simulink model "sm_boom_lift_crawler_abstract_flex_boom"  (R2026a)
settings: Solver=ode23t  StopTime=operator_seq.StopTime  FixedStep=2e-2  MaxStep=2  AbsTol=1e-3
PreLoadFcn:
  | sm_boom_lift_crawler_settest('full test')
StartFcn:
  | tic;
StopFcn:
  | Elapsed_Sim_Time = toc;
  | %disp(['Elapsed Sim Time = ' num2str(Elapsed_Sim_Time)]);
undefined symbols (not defined in the file or in its folder): b, BasketR, Boom, Chassis, Extend, FL, FR, Jib, LevelM, LevelS, Lift, operator_seq, OutFL, OutFR, OutRL, OutRR, RL, RR, Tilt, TrackL, TrackR, Turret, X, Y, Z
libraries: sm_lib x67, sm_boom_lift_crawler_lib x22, nesl_utility x15, sm_boom_lift_crawler_lib_boom x5, sm_boom_lift_crawler_lib_control x1, sm_boom_lift_crawler_lib_chassis x1
(part 1 of 5)
Description:
  | Boom Lift Crawler with Flexible Boom
  | 
  | Copyright 2020-2026 The MathWorks, Inc.
settings Model: PacingRate=0.100000  Creator=smiller  LastModifiedBy=smiller
settings DataIOCC: SignalLoggingName=logsout_sm_boom_lift_crawler
settings SimscapeCC: SimscapeNominalValues="[{\"value\":\"1\",\"unit\":\"A\"},{\"value\":\"nomval_psi\",\"unit\":\"psi\"},{\"value\":\"1\",\"unit\":\"cm^2\"},{\"value\":\"nomval_cmv3_s\",\"unit\":\"cm^3/s\"},{\"value\":\"1\",\"unit\":\"kJ/kg\"},{\"value\":\"1\",\"unit\":\"kW\"},{\"value\":\"1\",\"unit\":\"l\"},{\"value\":\"nomval_N\",\"unit\":\"N\"},{\"value\":\"nomval_Nm\",\"unit\":\"N*m\"},{\"value\":\"1\",\"unit\":\"V\"}]"  SimscapeLogName=simlog_sm_boom_lift_crawler  SimscapeLogLimitData=off  SimscapeLogDataHistory=5000.0  SimscapeOperatingPoint=op_hold15Sec_FULL
settings DiagnosticsConfigSet: SimMechanicsConflictingReferenceFrames=none  SimMechanicsRigidlyBoundBlock=none
settings ExplorerConfigSet: InternalSimMechanicsExplorerSettings="<ExplorerConfiguration><canonicalview>default</canonicalview><AnimationSetting><BasePlaybackSpeed>1.0</BasePlaybackSpeed><PlaybackSpeedFactor>1.0</PlaybackSpeedFactor></AnimationSetting><TilePanel><TileInfo><Tiles Columns=\"2\" Count=\"2\" Rows=\"1\"><Column Weight=\"0.4\"/><Column Weight=\"0.6\"/><Row Weight=\"1\"/><Tile Height=\"1\" Width=\"1\" X=\"0\" Y=\"0\"/><Tile Height=\"1\" Width=\"1\" X=\"1\" Y=\"0\"/></Tiles></TileInfo><SceneInfo><SceneViewer><BGColor><R>1</R><G>1</G><B>1</B></BGColor><Camera><DoPerspective>on</DoPerspective><Position><X>0.861797228389737158</X><Y>15.4087919652116785</Y><Z>1.5985929178525955</Z></Position><Center><X>0.688433827393987063</X><Y>14.4239340408412708</Y><Z>1.59859291785259594</Z></Center><Up><X>0</X><Y>0</Y><Z>1</Z></Up><ViewLimDist>1</ViewLimDist><YLim>0.466307658154998583</YLim><XLim>0.206102832333701025</XLim></Camera></SceneViewer><SceneViewer><BGColor><R>1</R><G>1</G><B>1</B></BGColor><Camera><DoPerspective>off</DoPerspective><Position><X>-13.0744225167074219</X><Y>9.83182144578760031</Y><Z>7.16198046954759793</Z></Position><Center><X>1.63071735726949996</X><Y>4.41437199856754514</Y><Z>7.1529177327451432</Z></Center><Up><X>0</X><Y>0</Y><Z>1</Z></Up><ViewLimDist>1</ViewLimDist><YLim>15.4925512172975477</YLim><XLim>10.3283674781983645</XLim></Camera></SceneViewer></SceneInfo></TilePanel><MechEditorPanel><Cameras><Camera><Id>Camera8</Id><Value><Name>Extend_Knuckle</Name><NativeCamera><PositionTrackingFeature>Lift.Boom.Arms.Telescope.Extend_Cylinder.Transform_Camera_Extend_Knuckle.F</PositionTrackingFeature><CenterTrackingFeature>Lift.Boom.Arms.Telescope.Extend_Cylinder.Transform_Camera_Extend_Knuckle.F</CenterTrackingFeature><UpVectorTrackingFeature>Lift.Boom.Arms.Telescope.Extend_Cylinder.Transform_Camera_Extend_Knuckle.F</UpVectorTrackingFeature><CenterTrackingOrigin>off</CenterTrackingOrigin><CenterTrackingDirection>-X</CenterTrackingDirection><UpVectorTrackingDirection>-Y</UpVectorTrackingDirection></NativeCamera></Value></Camera><Camera><Id>Camera9</Id><Value><Name>Extend_Basket</Name><NativeCamera><PositionTrackingFeature>Lift.Boom.Arms.Telescope.Extend_Cylinder.Transform_Camera_Extend_Basket.F</PositionTrackingFeature><CenterTrackingFeature>Lift.Boom.Arms.Telescope.Extend_Cylinder.Transform_Camera_Extend_Basket.F</CenterTrackingFeature><UpVectorTrackingFeature>Lift.Boom.Arms.Telescope.Extend_Cylinder.Transform_Camera_Extend_Basket.F</UpVectorTrackingFeature><CenterTrackingOrigin>off</CenterTrackingOrigin><CenterTrackingDirection>+X</CenterTrackingDirection><UpVectorTrackingDirection>+Y</UpVectorTrackingDirection></NativeCamera></Value></Camera><Camera><Id>Camera10</Id><Value><Name>Basket_Rotate</Name><NativeCamera><PositionTrackingFeature>Lift.Boom.Basket.Basket_Rotate.Bracket.Reference_Camera_Basket_Rotate_L.R</PositionTrackingFeature><CenterTrackingFeature>Lift.Boom.Basket.Basket_Rotate.Bracket.Reference_Camera_Basket_Rotate_L.R</CenterTrackingFeature><UpVectorTrackingFeature>Mech_Config.World.W</UpVectorTrackingFeature><CenterTrackingOrigin>off</CenterTrackingOrigin><CenterTrackingDirection>-X</CenterTrackingDirection><UpVectorTrackingDirection>+Z</UpVectorTrackingDirection></NativeCamera></Value></Camera><Camera><Id>Camera11</Id><Value><Name>Tilt_Knuckle</Name><NativeCamera><PositionTrackingFeature>Lift.Boom.Arms.Tower.Upper_Knuckle.Reference_Knuckle_Cam.R</PositionTrackingFeature><CenterTrackingFeature>Lift.Boom.Arms.Tower.Upper_Knuckle.Reference_Knuckle_Cam.R</CenterTrackingFeature><UpVectorTrackingFeature>Mech_Config.World.W</UpVectorTrackingFeature><CenterTrackingOrigin>off</CenterTrackingOrigin><CenterTrackingDirection>+Z</CenterTrackingDirection><UpVectorTrackingDirection>+Z</UpVectorTrackingDirection></NativeCamera></Value></Camera><Camera><Id>Camera12</Id><Value><Name>Full Test</Name><NativeCamera><PositionKeyframeSet><Keyframe><Time>0</Time><Value><X>-12.242458171438994</X><Y>-0.1433452642095574</Y><Z>4.1505972342390427</Z></Value></Keyframe><Keyframe><Time>69.026826430124729</Time><Value><X>-14.974593328379619</X><Y>0.0056652615564253064</Y><Z>5.3389029552684786</Z></Value></Keyframe><Keyframe><Time>110.29539843687829</Time><Value><X>-21.00761369699504</X><Y>-0.0057417156870510078</Y><Z>8.0689402037867488</Z></Value></Keyframe><Keyframe><Time>140.70430157635164</Time><Value><X>-31.272784439198116</X><Y>-2.5583130214499052e-10</Y><Z>12.723321478963756</Z></Value></Keyframe><Keyframe><Time>181.77628976806102</Time><Value><X>-31.272784439198116</X><Y>-2.5583130214499052e-10</Y><Z>12.723321478963756</Z></Value></Keyframe><Keyframe><Time>208.0087867386398</Time><Value><X>-23.351505250921551</X><Y>-2.5583182919801497e-10</Y><Z>9.1371534281977738</Z></Value></Keyframe><Keyframe><Time>243.06358572448306</Time><Value><X>-16.577121762622586</X><Y>-2.5583144573665537e-10</Y><Z>6.0702143126734844</Z></Value></Keyframe><Keyframe><Time>273.3415757110605</Time><Value><X>-16.577121762622586</X><Y>-2.5583144573665537e-10</Y><Z>6.0702143126734844</Z></Value></Keyframe><Keyframe><Time>321.2447002217541</Time><Value><X>-13.690590902490033</X><Y>0.01787769923724114</Y><Z>4.7891626503614262</Z></Value></Keyframe><Keyframe><Time>350</Time><Value><X>-13.690590902490033</X><Y>0.01787769923724114</Y><Z>4.7891626503614262</Z></Value></Keyframe></PositionKeyframeSet><CenterKeyframeSet><Keyframe><Time>0</Time><Value><X>-4.621228999686064</X><Y>-0.1433452642095574</Y><Z>4.1505972342390436</Z></Value></Keyframe><Keyframe><Time>69.026826430124729</Time><Value><X>-0.17395018713353672</X><Y>0.0056652615564253064</Y><Z>5.3389029552684786</Z></Value></Keyframe><Keyframe><Time>110.29539843687829</Time><Value><X>-9.0038066291239502</X><Y>-0.0057417156870549491</Y><Z>8.0689402037867524</Z></Value></Keyframe><Keyframe><Time>140.70430157635164</Time><Value><X>-14.136391845814327</X><Y>-2.5583979379462107e-10</Y><Z>12.72332147896376</Z></Value></Keyframe><Keyframe><Time>181.77628976806102</Time><Value><X>-2.3429975002054775</X><Y>-2.5584563781180217e-10</Y><Z>12.723321478963761</Z></Value></Keyframe><Keyframe><Time>208.0087867386398</Time><Value><X>-10.17575261115104</X><Y>-2.5583801743778167e-10</Y><Z>9.1371534281977755</Z></Value></Keyframe><Keyframe><Time>243.06358572448306</Time><Value><X>-0.54476849060194255</X><Y>-2.5583897563257738e-10</Y><Z>6.0702143126734844</Z></Value></Keyframe><Keyframe><Time>273.3415757110605</Time><Value><X>-0.11057247639663359</X><Y>-2.5583917956089291e-10</Y><Z>6.0702143126734844</Z></Value></Keyframe><Keyframe><Time>321.2447002217541</Time><Value><X>-5.3452949964231387</X><Y>0.017877699237237366</Y><Z>4.7891626503614253</Z></Value></Keyframe><Keyframe><Time>350</Time><Value><X>-5.3452949964231387</X><Y>0.017877699237237366</Y><Z>4.7891626503614253</Z></Value></Keyframe></CenterKeyframeSet><UpVectorKeyframeSet><Keyframe><Time>0</Time><Value><X>0</X><Y>0</Y><Z>1</Z></Value></Keyframe><Keyframe><Time>69.026826430124729</Time><Value><X>0</X><Y>0</Y><Z>1</Z></Value></Keyframe><Keyframe><Time>110.29539843687829</Time><Value><X>0</X><Y>0</Y><Z>1</Z></Value></Keyframe><Keyframe><Time>140.70430157635164</Time><Value><X>0</X><Y>0</Y><Z>1</Z></Value></Keyframe><Keyframe><Time>181.77628976806102</Time><Value><X>-2.0731981129868445e-16</X><Y>1.0273382740432149e-31</Y><Z>1</Z></Value></Keyframe><Keyframe><Time>208.0087867386398</Time><Value><X>1.4663775813922931e-57</X><Y>2.9591920320379324e-42</Y><Z>1</Z></Value></Keyframe><Keyframe><Time>243.06358572448306</Time><Value><X>1.3898401336634517e-57</X><Y>2.9591920320379324e-42</Y><Z>1</Z></Value></Keyframe><Keyframe><Time>273.3415757110605</Time><Value><X>1.3898401336605064e-57</X><Y>2.9591920320379324e-42</Y><Z>1</Z></Value></Keyframe><Keyframe><Time>321.2447002217541</Time><Value><X>1.3198478700492623e-57</X><Y>2.9591920320379324e-42</Y><Z>1</Z></Value></Keyframe><Keyframe><Time>350</Time><Value><X>1.0642863113510858e-16</X><Y>-4.813997747953607e-32</Y><Z>1</Z></Value></Keyframe></UpVectorKeyframeSet></NativeCamera></Value></Camera><Camera><Id>Camera13</Id><Value><Name>View_Basket_World</Name><NativeCamera><PositionTrackingFeature>Lift.Boom.Basket.Basket.Reference_Basket_Cam.R</PositionTrackingFeature><CenterTrackingFeature>Mech_Config.World.W</CenterTrackingFeature><UpVectorTrackingFeature>Lift.Boom.Basket.Basket.Reference_Basket_Cam.R</UpVectorTrackingFeature><CenterTrackingOrigin>on</CenterTrackingOrigin><UpVectorTrackingDirection>+Y</UpVectorTrackingDirection></NativeCamera></Value></Camera><Camera><Id>Camera14</Id><Value><Name>View_Worm_Drive</Name><NativeCamera><PositionTrackingFeature>Lift.Boom.Turret.Case.Reference_Worm_Cam.R</PositionTrackingFeature><CenterTrackingFeature>Lift.Boom.Turret.Case.Transform_Worm_Cam.B</CenterTrackingFeature><UpVectorTrackingFeature>Mech_Config.World.W</UpVectorTrackingFeature><CenterTrackingOrigin>on</CenterTrackingOrigin><UpVectorTrackingDirection>+Z</UpVectorTrackingDirection></NativeCamera></Value></Camera><Camera><Id>Camera15</Id><Value><Name>Extend_Retract_Pulley</Name><NativeCamera><PositionTrackingFeature>Lift.Boom.Arms.Telescope.Extend_Cylinder.Reference_Camera_Retract_Pulley.R</PositionTrackingFeature><CenterTrackingFeature>Lift.Boom.Arms.Telescope.Extend_Cylinder.Reference_Camera_Retract_Pulley.R</CenterTrackingFeature><UpVectorTrackingFeature>Lift.Boom.Arms.Telescope.Extend_Cylinder.Reference_Camera_Retract_Pulley.R</UpVectorTrackingFeature><CenterTrackingOrigin>off</CenterTrackingOrigin><CenterTrackingDirection>+Y</CenterTrackingDirection><UpVectorTrackingDirection>+Z</UpVectorTrackingDirection></NativeCamera></Value></Camera><Camera><Id>Camera16</Id><Value><Name>Extend_Extend_Pulley</Name><NativeCamera><PositionTrackingFeature>Lift.Boom.Arms.Telescope.Extend_Cylinder.Reference_Camera_Extend_Pulley.R</PositionTrackingFeature><CenterTrackingFeature>Lift.Boom.Arms.Telescope.Extend_Cylinder.Reference_Camera_Extend_Pulley.R</CenterTrackingFeature><UpVectorTrackingFeature>Lift.Boom.Arms.Telescope.Extend_Cylinder.Reference_Camera_Extend_Pulley.R</UpVectorTrackingFeature><CenterTrackingOrigin>off</CenterTrackingOrigin><CenterTrackingDirection>+Z</CenterTrackingDirection><UpVectorTrackingDirection>-Y</UpVectorTrackingDirection></NativeCamera></Value></Camera><Camera><Id>Camera17</Id><Value><Name>Jib</Name><NativeCamera><PositionTrackingFeature>Lift.Boom.Basket.Jib.Jib_Mount.Reference_Camera_Basket_Jib.R</PositionTrackingFeature><CenterTrackingFeature>Lift.Boom.Basket.Jib.Jib_Mount.Reference_Camera_Basket_Jib.R</CenterTrackingFeature><UpVectorTrackingFeature>Mech_Config.World.W</UpVectorTrackingFeature><CenterTrackingOrigin>off</CenterTrackingOrigin><CenterTrackingDirection>-X</CenterTrackingDirection><UpVectorTrackingDirection>+Z</UpVectorTrackingDirection></NativeCamera></Value></Camera><Camera><Id>Camera18</Id><Value><Name>Boom Align</Name><NativeCamera><PositionTrackingFeature>Lift.Chassis.Frame.Reference_Camera_Boom_Align_R</PositionTrackingFeature><CenterTrackingFeature>Lift.Chassis.Frame.Reference_Camera_Boom_Align_R</CenterTrackingFeature><UpVectorTrackingFeature>Lift.Chassis.Frame.Reference_Camera_Boom_Align_R</UpVectorTrackingFeature><CenterTrackingOrigin>off</CenterTrackingOrigin><CenterTrackingDirection>+Y</CenterTrackingDirection><UpVectorTrackingDirection>+Z</UpVectorTrackingDirection></NativeCamera></Value></Camera><Camera><Id>Camera19</Id><Value><Name>Basket_Boom</Name><NativeCamera><PositionTrackingFeature>Lift.Boom.Arms.Camera_Boom_Basket.Reference_Basket_Boom_Cam.R</PositionTrackingFeature><CenterTrackingFeature>Lift.Boom.Arms.Camera_Boom_Basket.Reference_Basket_Boom_Cam.R</CenterTrackingFeature><UpVectorTrackingFeature>Mech_Config.World.W</UpVectorTrackingFeature><CenterTrackingOrigin>off</CenterTrackingOrigin><CenterTrackingDirection>+X</CenterTrackingDirection><UpVectorTrackingDirection>+Z</UpVectorTrackingDirection></NativeCamera></Value></Camera></Cameras><GfxPanelCameraMap><MapElement CameraMLId=\"Camera19\" GfxPanelIndex=\"0\"/></GfxPanelCameraMap><VideoCreator><PlaybackSpeedRatio>1.0</PlaybackSpeedRatio><FrameRate>30</FrameRate><VideoFormat>MPEG-4</VideoFormat><FrameSize>auto</FrameSize></VideoCreator></MechEditorPanel></ExplorerConfiguration>"

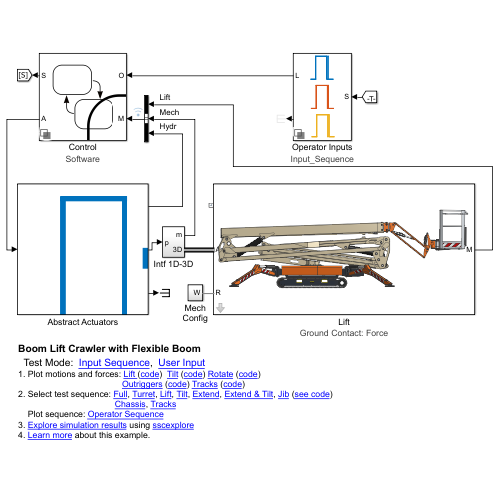
[thumbnail: Simulink's stored preview of the top-level diagram]
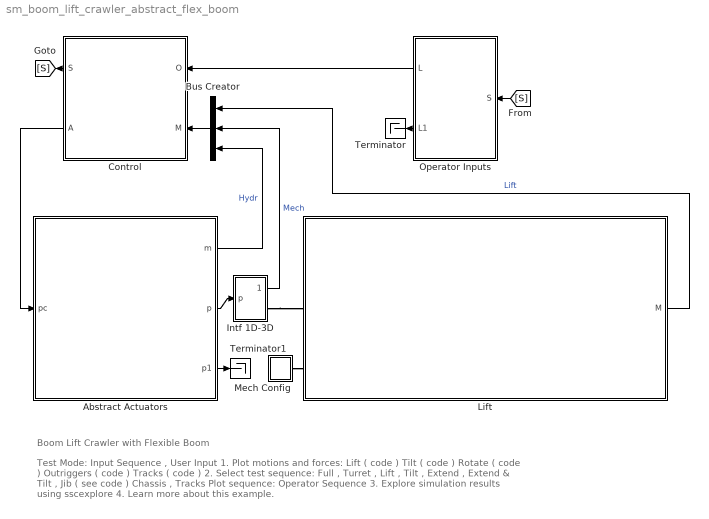
== system sm_boom_lift_crawler_abstract_flex_boom ==
  note: Test Mode: Input Sequence , User Input
      | 1. Plot motions and forces: Lift ( code ) Tilt ( code ) Rotate ( code )
      | Outriggers ( code ) Tracks ( code )
      | 2. Select test sequence: Full , Turret , Lift , Tilt , Extend , Extend & Tilt , Jib ( see code )
      | Chassis , Tracks
      | Plot sequence: Operator Sequence
      | 3. Explore simulation results using sscexplore
      | 4. Learn more about this example.
  note: Boom Lift Crawler with Flexible Boom
  Abstract Actuators : Subsystem  VariantControl=Controller_Inputs
      mask Display: image('sm_boom_lift_crawler_logic_to_motion_seq.svg');
  Bus Creator : BusCreator  Inputs=3
  Control : Subsystem  Variant=on  VariantControlMode=label  VariantControl=Variant1  LabelModeActiveChoice=Software
      settings: AttributesFormatString=%<LabelModeActiveChoice>
      mask Display:
      | blk = sm_boom_lift_activeVariantBlock(gcb);
      | eval(get_param(blk, 'MaskDisplay'));
  Intf 1D-3D : Subsystem
  Lift : Subsystem  mask{popup_gnd_outr=Force}
      mask prompts: popup_gnd_outr "Ground Contact (Outrigger)"
      mask init:
      | set_param([gcb '/Ground Contact Pads'],'LabelModeActiveChoice',get_param(gcb,'popup_gnd_outr'));
      settings: AttributesFormatString=Ground Contact: %<popup_gnd_outr>
      mask TypeOptions popup_gnd_outr: Force | Constraint
      mask Display: image('sm001_2x1_v2.svg');
  Mech Config : Subsystem
  Operator Inputs : Subsystem  Variant=on  VariantControlMode=label  VariantControl=Variant1  LabelModeActiveChoice=Input_Sequence
      settings: AttributesFormatString=%<LabelModeActiveChoice>
      mask Display:
      | blk = sm_boom_lift_activeVariantBlock(gcb);
      | eval(get_param(blk, 'MaskDisplay'));
  Terminator : Terminator
  Terminator1 : Terminator
  wires:
  Intf 1D-3D/1(m) -> Bus Creator/2  "Mech"
  Bus Creator/1 -> Control/2(M)
  Lift/1(M) -> Bus Creator/1  "Lift"
  Control/2(A) -> Abstract Actuators/1(pc)
  Abstract Actuators/2(p) -> Intf 1D-3D/1(p)
  Abstract Actuators/3(p1) -> Terminator1/1
  Abstract Actuators/1(m) -> Bus Creator/3  "Hydr"
  Operator Inputs/1(L) -> Control/1(O)
  Operator Inputs/2(L1) -> Terminator/1
  Control/1(S) -> [S]
  [S] -> Operator Inputs/1(S)
  connections:
  Mech Config/LConn1 -- Lift/LConn3
  Intf 1D-3D/RConn1 -- Lift/LConn2

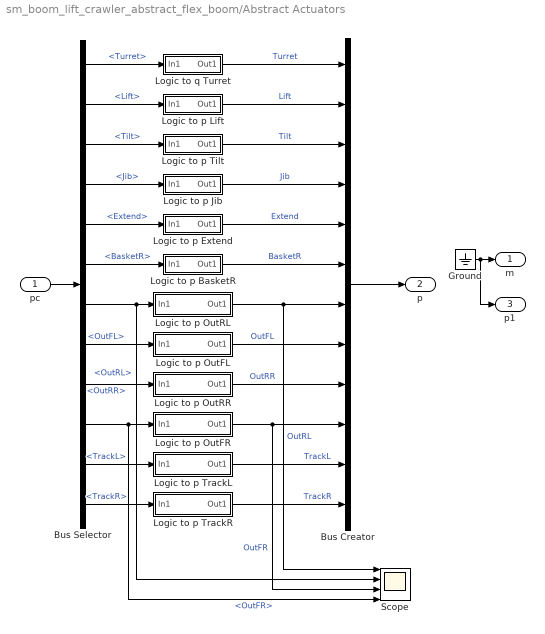
== system sm_boom_lift_crawler_abstract_flex_boom/Abstract Actuators ==
  pc : Inport
  Bus Creator : BusCreator  Inputs=12
  Bus Selector : BusSelector  OutputSignals=Turret,Lift,Tilt,Jib,Extend,BasketR,OutRL,OutFL,OutRR,OutFR,TrackL,TrackR
  Ground : Ground
  Logic to p BasketR : Subsystem
  Logic to p Extend : Subsystem
  Logic to p Jib : Subsystem
  Logic to p Lift : Subsystem
  Logic to p OutFL : Subsystem
  Logic to p OutFR : Subsystem
  Logic to p OutRL : Subsystem
  Logic to p OutRR : Subsystem
  Logic to p Tilt : Subsystem
  Logic to p TrackL : Subsystem
  Logic to p TrackR : Subsystem
  Logic to q Turret : Subsystem
  Scope : Scope  NumInputPorts=4
      settings: ActiveDisplayYMinimum=12.92005  ActiveDisplayYMaximum=13.76598
  m : Outport
  p : Outport  Port=2
  p1 : Outport  Port=3
  wires:
  Ground/1 -> m/1, p1/1
  pc/1 -> Bus Selector/1
  Bus Selector/12 -> Logic to p TrackR/1(In1)  "<TrackR>"
  Bus Selector/11 -> Logic to p TrackL/1(In1)  "<TrackL>"
  Bus Selector/2 -> Logic to p Lift/1(In1)  "<Lift>"
  Logic to p TrackL/1(Out1) -> Bus Creator/11  "TrackL"
  Bus Selector/6 -> Logic to p BasketR/1(In1)  "<BasketR>"
  Bus Selector/5 -> Logic to p Extend/1(In1)  "<Extend>"
  Bus Creator/1 -> p/1
  Bus Selector/1 -> Logic to q Turret/1(In1)  "<Turret>"
  Bus Selector/7 -> Scope/2, Logic to p OutRL/1(In1)  "<OutRL>"
  Bus Selector/3 -> Logic to p Tilt/1(In1)  "<Tilt>"
  Logic to p Lift/1(Out1) -> Bus Creator/2  "Lift"
  Bus Selector/8 -> Logic to p OutFL/1(In1)  "<OutFL>"
  Bus Selector/4 -> Logic to p Jib/1(In1)  "<Jib>"
  Logic to p TrackR/1(Out1) -> Bus Creator/12  "TrackR"
  Bus Selector/9 -> Logic to p OutRR/1(In1)  "<OutRR>"
  Bus Selector/10 -> Scope/4, Logic to p OutFR/1(In1)  "<OutFR>"
  Logic to q Turret/1(Out1) -> Bus Creator/1  "Turret"
  Logic to p OutRL/1(Out1) -> Scope/1, Bus Creator/7  "OutRL"
  Logic to p OutFL/1(Out1) -> Bus Creator/8  "OutFL"
  Logic to p OutRR/1(Out1) -> Bus Creator/9  "OutRR"
  Logic to p OutFR/1(Out1) -> Scope/3, Bus Creator/10  "OutFR"
  Logic to p Tilt/1(Out1) -> Bus Creator/3  "Tilt"
  Logic to p Jib/1(Out1) -> Bus Creator/4  "Jib"
  Logic to p Extend/1(Out1) -> Bus Creator/5  "Extend"
  Logic to p BasketR/1(Out1) -> Bus Creator/6  "BasketR"

== system sm_boom_lift_crawler_abstract_flex_boom/Control ==
  O : Inport
  M : Inport  Port=2
  Direct : Subsystem  VariantControl=Direct
      mask Display: image('sm_boom_lift_crawler_control_direct.svg');
  Software : sm_boom_lift_crawler_lib_control/Software  SystemSampleTime=-1  VariantControl=Software  VariantActivationTime=update diagram  EmptyChoice=off  PassThrough=off  PassThroughVariantControl=(default)  EmptyChoiceVariantControl=(default)  AllowFlexibleInterface=on  Latency=0  AutoFrameSizeCalculation=off
  S : Outport
  A : Outport  Port=2

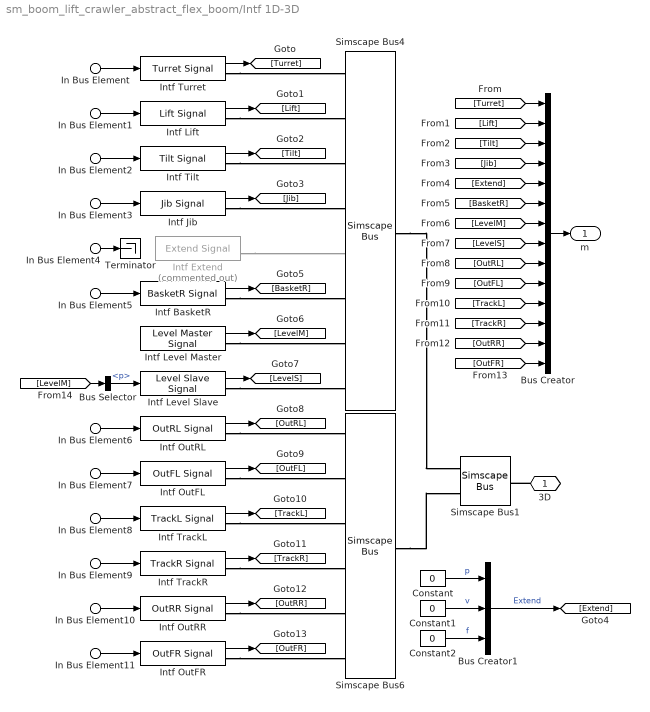
== system sm_boom_lift_crawler_abstract_flex_boom/Intf 1D-3D ==
  In Bus Element : Inport  PortName=p  Element=Turret
  In Bus Element1 : Inport  PortName=p  Element=Lift
  In Bus Element2 : Inport  PortName=p  Element=Tilt
  In Bus Element3 : Inport  PortName=p  Element=Jib
  In Bus Element4 : Inport  PortName=p  Element=Extend
  In Bus Element5 : Inport  PortName=p  Element=BasketR
  In Bus Element6 : Inport  PortName=p  Element=OutRL
  In Bus Element7 : Inport  PortName=p  Element=OutFL
  In Bus Element8 : Inport  PortName=p  Element=TrackL
  In Bus Element9 : Inport  PortName=p  Element=TrackR
  In Bus Element10 : Inport  PortName=p  Element=OutRR
  In Bus Element11 : Inport  PortName=p  Element=OutFR
  Bus Creator : BusCreator  Inputs=14
  Bus Creator1 : BusCreator  Inputs=3
  Bus Selector : BusSelector  OutputSignals=p
  Constant : Constant  Value=0
  Constant1 : Constant  Value=0
  Constant2 : Constant  Value=0
  Intf BasketR : sm_boom_lift_crawler_lib/BasketR Signal  SystemSampleTime=-1  VariantActivationTime=update diagram  EmptyChoice=off  PassThrough=off  PassThroughVariantControl=(default)  EmptyChoiceVariantControl=(default)  AllowFlexibleInterface=on  Latency=0  AutoFrameSizeCalculation=off
  Intf Extend : sm_boom_lift_crawler_lib/Extend Signal  Commented=on  SystemSampleTime=-1  VariantActivationTime=update diagram  EmptyChoice=off  PassThrough=off  PassThroughVariantControl=(default)  EmptyChoiceVariantControl=(default)  AllowFlexibleInterface=on  Latency=0  AutoFrameSizeCalculation=off
  Intf Jib : sm_boom_lift_crawler_lib/Jib Signal  SystemSampleTime=-1  VariantActivationTime=update diagram  EmptyChoice=off  PassThrough=off  PassThroughVariantControl=(default)  EmptyChoiceVariantControl=(default)  AllowFlexibleInterface=on  Latency=0  AutoFrameSizeCalculation=off
  Intf Level Master : sm_boom_lift_crawler_lib/Level Master Signal  SystemSampleTime=-1  VariantActivationTime=update diagram  EmptyChoice=off  PassThrough=off  PassThroughVariantControl=(default)  EmptyChoiceVariantControl=(default)  AllowFlexibleInterface=on  Latency=0  AutoFrameSizeCalculation=off
  Intf Level Slave : sm_boom_lift_crawler_lib/Level Slave Signal  SystemSampleTime=-1  VariantActivationTime=update diagram  EmptyChoice=off  PassThrough=off  PassThroughVariantControl=(default)  EmptyChoiceVariantControl=(default)  AllowFlexibleInterface=on  Latency=0  AutoFrameSizeCalculation=off
  Intf Lift : sm_boom_lift_crawler_lib/Lift Signal  SystemSampleTime=-1  VariantActivationTime=update diagram  EmptyChoice=off  PassThrough=off  PassThroughVariantControl=(default)  EmptyChoiceVariantControl=(default)  AllowFlexibleInterface=on  Latency=0  AutoFrameSizeCalculation=off
  Intf OutFL : sm_boom_lift_crawler_lib/OutFL Signal  SystemSampleTime=-1  VariantActivationTime=update diagram  EmptyChoice=off  PassThrough=off  PassThroughVariantControl=(default)  EmptyChoiceVariantControl=(default)  AllowFlexibleInterface=on  Latency=0  AutoFrameSizeCalculation=off
  Intf OutFR : sm_boom_lift_crawler_lib/OutFR Signal  SystemSampleTime=-1  VariantActivationTime=update diagram  EmptyChoice=off  PassThrough=off  PassThroughVariantControl=(default)  EmptyChoiceVariantControl=(default)  AllowFlexibleInterface=on  Latency=0  AutoFrameSizeCalculation=off
  Intf OutRL : sm_boom_lift_crawler_lib/OutRL Signal  SystemSampleTime=-1  VariantActivationTime=update diagram  EmptyChoice=off  PassThrough=off  PassThroughVariantControl=(default)  EmptyChoiceVariantControl=(default)  AllowFlexibleInterface=on  Latency=0  AutoFrameSizeCalculation=off
  Intf OutRR : sm_boom_lift_crawler_lib/OutRR Signal  SystemSampleTime=-1  VariantActivationTime=update diagram  EmptyChoice=off  PassThrough=off  PassThroughVariantControl=(default)  EmptyChoiceVariantControl=(default)  AllowFlexibleInterface=on  Latency=0  AutoFrameSizeCalculation=off
  Intf Tilt : sm_boom_lift_crawler_lib/Tilt Signal  SystemSampleTime=-1  VariantActivationTime=update diagram  EmptyChoice=off  PassThrough=off  PassThroughVariantControl=(default)  EmptyChoiceVariantControl=(default)  AllowFlexibleInterface=on  Latency=0  AutoFrameSizeCalculation=off
  Intf TrackL : sm_boom_lift_crawler_lib/TrackL Signal  SystemSampleTime=-1  VariantActivationTime=update diagram  EmptyChoice=off  PassThrough=off  PassThroughVariantControl=(default)  EmptyChoiceVariantControl=(default)  AllowFlexibleInterface=on  Latency=0  AutoFrameSizeCalculation=off
  Intf TrackR : sm_boom_lift_crawler_lib/TrackR Signal  SystemSampleTime=-1  VariantActivationTime=update diagram  EmptyChoice=off  PassThrough=off  PassThroughVariantControl=(default)  EmptyChoiceVariantControl=(default)  AllowFlexibleInterface=on  Latency=0  AutoFrameSizeCalculation=off
  Intf Turret : sm_boom_lift_crawler_lib/Turret Signal  SystemSampleTime=-1  VariantActivationTime=update diagram  EmptyChoice=off  PassThrough=off  PassThroughVariantControl=(default)  EmptyChoiceVariantControl=(default)  AllowFlexibleInterface=on  Latency=0  AutoFrameSizeCalculation=off
  Simscape Bus1 : SimscapeBus  HierarchyStrings=Boom;Chassis
  Simscape Bus4 : SimscapeBus  HierarchyStrings=Turret;Lift;Tilt;Jib;Extend;BasketR;LevelM;LevelS
  Simscape Bus6 : SimscapeBus  HierarchyStrings=OutRL;OutFL;TrackL;TrackR;OutRR;OutFR
  Terminator : Terminator
  3D : PMIOPort  Side=Right
  m : Outport
  wires:
  Intf OutFR/1 -> [OutFR]
  Intf OutRR/1 -> [OutRR]
  Intf TrackR/1 -> [TrackR]
  Intf TrackL/1 -> [TrackL]
  Intf OutFL/1 -> [OutFL]
  Intf OutRL/1 -> [OutRL]
  Intf Level Slave/1 -> [LevelS]
  Intf Level Master/1 -> [LevelM]
  Intf BasketR/1 -> [BasketR]
  Intf Jib/1 -> [Jib]
  Intf Tilt/1 -> [Tilt]
  Intf Lift/1 -> [Lift]
  Intf Turret/1 -> [Turret]
  [OutFR] -> Bus Creator/14
  [OutRR] -> Bus Creator/13
  [Extend] -> Bus Creator/5
  [OutRL] -> Bus Creator/9
  [TrackL] -> Bus Creator/11
  [LevelM] -> Bus Creator/7
  [Turret] -> Bus Creator/1
  [OutFL] -> Bus Creator/10
  [Tilt] -> Bus Creator/3
  [Lift] -> Bus Creator/2
  [TrackR] -> Bus Creator/12
  [LevelS] -> Bus Creator/8
  Bus Creator/1 -> m/1
  [Jib] -> Bus Creator/4
  [BasketR] -> Bus Creator/6
  Bus Selector/1 -> Intf Level Slave/1  "<p>"
  [LevelM] -> Bus Selector/1
  In Bus Element/1 -> Intf Turret/1
  In Bus Element1/1 -> Intf Lift/1
  In Bus Element2/1 -> Intf Tilt/1
  In Bus Element3/1 -> Intf Jib/1
  In Bus Element4/1 -> Terminator/1
  In Bus Element5/1 -> Intf BasketR/1
  In Bus Element6/1 -> Intf OutRL/1
  In Bus Element7/1 -> Intf OutFL/1
  In Bus Element8/1 -> Intf TrackL/1
  In Bus Element9/1 -> Intf TrackR/1
  In Bus Element10/1 -> Intf OutRR/1
  In Bus Element11/1 -> Intf OutFR/1
  Constant2/1 -> Bus Creator1/3  "f"
  Constant1/1 -> Bus Creator1/2  "v"
  Bus Creator1/1 -> [Extend]  "Extend"
  Constant/1 -> Bus Creator1/1  "p"
  connections:
  Intf OutRR/RConn1 -- Simscape Bus6/LConn5
  Intf OutFR/RConn1 -- Simscape Bus6/LConn6
  Intf TrackR/RConn1 -- Simscape Bus6/LConn4
  Intf TrackL/RConn1 -- Simscape Bus6/LConn3
  Intf OutRL/RConn1 -- Simscape Bus6/LConn1
  Intf OutFL/RConn1 -- Simscape Bus6/LConn2
  Simscape Bus6/RConn1 -- Simscape Bus1/LConn2
  Intf Level Slave/RConn1 -- Simscape Bus4/LConn8
  Intf Level Master/RConn1 -- Simscape Bus4/LConn7
  Intf BasketR/RConn1 -- Simscape Bus4/LConn6
  Intf Extend/RConn1 -- Simscape Bus4/LConn5
  Intf Jib/RConn1 -- Simscape Bus4/LConn4
  Intf Tilt/RConn1 -- Simscape Bus4/LConn3
  Intf Lift/RConn1 -- Simscape Bus4/LConn2
  Intf Turret/RConn1 -- Simscape Bus4/LConn1
  Simscape Bus4/RConn1 -- Simscape Bus1/LConn1
  3D/RConn1 -- Simscape Bus1/RConn1

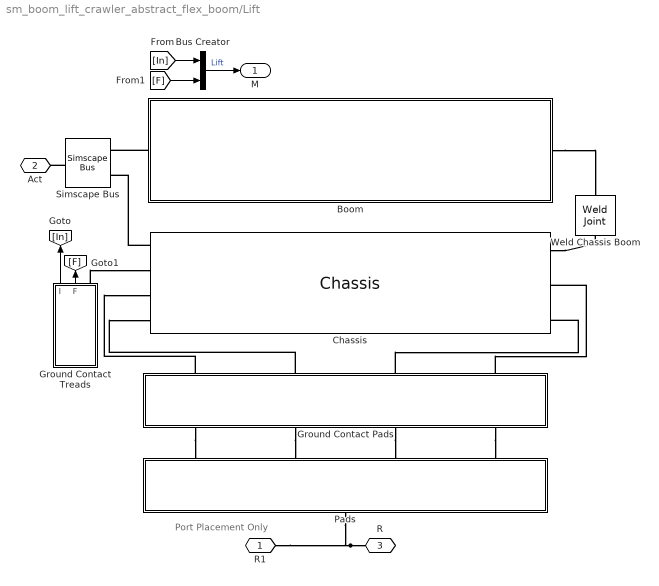
== system sm_boom_lift_crawler_abstract_flex_boom/Lift ==
  note: Port
      | Placement
      | Only
  Boom : Subsystem
      mask Display: image('sm002.svg');
  Bus Creator : BusCreator  Inputs=2
  Chassis : sm_boom_lift_crawler_lib_chassis/Chassis  SystemSampleTime=-1  VariantActivationTime=update diagram  EmptyChoice=off  PassThrough=off  PassThroughVariantControl=(default)  EmptyChoiceVariantControl=(default)  AllowFlexibleInterface=on  Latency=0  AutoFrameSizeCalculation=off
  Ground Contact Pads : Subsystem  Variant=on  VariantControlMode=label  VariantControl=Variant1  LabelModeActiveChoice=Force
      settings: AttributesFormatString=%<LabelModeActiveChoice>
      mask Display:
      | blk = sm_boom_lift_activeVariantBlock(gcb);
      | eval(get_param(blk, 'MaskDisplay'));
  Ground Contact Treads : Subsystem
      mask Display: image('sm_boom_lift_crawler_contact_track_floor.svg');
  Pads : Subsystem
      mask Display: image('sm004.svg');
  Simscape Bus : SimscapeBus  HierarchyStrings=Boom;Chassis
  Weld Chassis Boom : sm_lib/Joints/Weld Joint  JointMode=Normal  CompositeWrenchDir=FollowerOnBase  CompositeWrenchFrame=BaseFrame  SenseConstraintForce=off  SenseConstraintTorque=off  SenseTotalForce=off  SenseTotalTorque=off
  R1 : PMIOPort  Side=Left
  Act : PMIOPort  Port=2  Side=Left
  R : PMIOPort  Port=3  Side=Left
  M : Outport
  wires:
  [F] -> Bus Creator/2
  [In] -> Bus Creator/1
  Ground Contact Treads/2(F) -> [F]
  Ground Contact Treads/1(I) -> [In]
  Bus Creator/1 -> M/1  "Lift"
  connections:
  Ground Contact Pads/RConn4 -- Chassis/RConn2
  Ground Contact Pads/RConn3 -- Chassis/RConn3
  Ground Contact Pads/RConn2 -- Chassis/LConn4
  Ground Contact Pads/RConn1 -- Chassis/LConn3
  Ground Contact Pads/LConn4 -- Pads/LConn4
  Ground Contact Pads/LConn3 -- Pads/LConn3
  Ground Contact Pads/LConn2 -- Pads/LConn2
  Ground Contact Pads/LConn1 -- Pads/LConn1
  R/RConn1 -- Pads/RConn1 -- R1/RConn1
  Ground Contact Treads/RConn1 -- Chassis/LConn2
  Simscape Bus/RConn1 -- Act/RConn1
  Chassis/LConn1 -- Simscape Bus/LConn2
  Boom/LConn1 -- Simscape Bus/LConn1
  Boom/RConn1 -- Weld Chassis Boom/RConn1
  Chassis/RConn1 -- Weld Chassis Boom/LConn1

== system sm_boom_lift_crawler_abstract_flex_boom/Mech Config ==
  Mechanism Configuration : sm_lib/Utilities/Mechanism Configuration  UniformGravity=Constant  GravityVector=[0 0 -9.80665]  GravityVectorUnits=m/s^2  LinearizationDelta=0.001  JointModeTransitionNonlinearIterations=2
  Solver Configuration : nesl_utility/Solver Configuration  PhysicalDomain=network_engine_domain  SubClassName=solver  LeftPortType=input  RightPortType=generic  Tones=[]  Harmonics=[]  SimulateNoise=off  Profile=off  UseLocalSampling=off  EnableSwitchedLinearOptims=on  FrequencyDomain=off  UseCCode=off  RelTol=0.001  AbsTol=1e-06  MinStep=1e-09  ToWorkspace=off  RevertToSquareIcSolve=off  NumHomotopyIterations=100  PhasorMode=off  PhasorModeNumHarmonics=1  ConsistencySolver=NEWTON_FTOL  CanonicalOrdering=UNORDERED  OptimizeIntermediates=UNOPTIMIZED  IndexReductionMethod=DerivativeReplacement  DoDC=off  ResidualTolerance=1e-9  ConsistencyTolSource=GLOBAL  ConsistencyAbsTol=0.001  ConsistencyRelTol=0.001  ConsistencyTolFactor=0.001  UseLocalSolver=off  LocalSolverChoice=NE_BACKWARD_EULER_ADVANCER  ResolveIndetEquations=on  FunctionEvalNumThread=1  LocalSolverSampleTime=2e-3  DoFixedCost=off  MaxNonlinIter=3  MaxModeIter=2  ComputeImpulses=off  ImpulseIterations=2  LinearAlgebra=auto  LinearAlgebraNumThread=0  EquationFormulation=NE_TIME_EF  DelaysMemoryBudget=1024  AutomaticFiltering=on  FilteringTimeConstant=0.001  PartitionStorageMethod=AS_NEEDED  PartitionMemoryBudget=1024  PartitionMethod=ROBUST  MultibodyUseLocalSolver=off  MultibodyLocalSolverChoice=ODE1  MultibodyLocalSolverSampleTime=0.001
  World : sm_lib/Frames and Transforms/World Frame
  W : PMIOPort  Side=Left
  connections:
  Solver Configuration/RConn1 -- W/RConn1 -- Mechanism Configuration/RConn1 -- World/RConn1

== system sm_boom_lift_crawler_abstract_flex_boom/Operator Inputs ==
  S : Inport
  Input Sequence : Subsystem  VariantControl=Input_Sequence
      mask Display: image('sm_boom_lift_crawler_operator_seq.svg');
  User Input : Subsystem  VariantControl=User_Input
      mask Display: image('sl001_2x3.svg');
  L : Outport
  L1 : Outport  Port=2

== system sm_boom_lift_crawler_abstract_flex_boom/Abstract Actuators/Logic to p BasketR ==
  In1 : Inport
  Gain : Gain  Gain=0.5450
  Integrator : Integrator  LimitOutput=on  UpperSaturationLimit=1.09  LowerSaturationLimit=0
  Out1 : Outport
  wires:
  Gain/1 -> Integrator/1
  In1/1 -> Gain/1
  Integrator/1 -> Out1/1

== system sm_boom_lift_crawler_abstract_flex_boom/Abstract Actuators/Logic to p Extend ==
  In1 : Inport
  Gain : Gain  Gain=0.1676
  Integrator : Integrator  InitialCondition=0.0063  LimitOutput=on  UpperSaturationLimit=3.86  LowerSaturationLimit=0
  Out1 : Outport
  wires:
  Integrator/1 -> Out1/1
  In1/1 -> Gain/1
  Gain/1 -> Integrator/1

== system sm_boom_lift_crawler_abstract_flex_boom/Abstract Actuators/Logic to p Jib ==
  In1 : Inport
  Gain : Gain  Gain=0.0373
  Integrator : Integrator  LimitOutput=on  UpperSaturationLimit=0.358  LowerSaturationLimit=0
  Out1 : Outport
  wires:
  Gain/1 -> Integrator/1
  In1/1 -> Gain/1
  Integrator/1 -> Out1/1

== system sm_boom_lift_crawler_abstract_flex_boom/Abstract Actuators/Logic to p Lift ==
  In1 : Inport
  Gain : Gain  Gain=0.0120
  Integrator : Integrator  LimitOutput=on  UpperSaturationLimit=0.57  LowerSaturationLimit=0
  Out1 : Outport
  wires:
  Gain/1 -> Integrator/1
  In1/1 -> Gain/1
  Integrator/1 -> Out1/1

== system sm_boom_lift_crawler_abstract_flex_boom/Abstract Actuators/Logic to p OutFL ==
  In1 : Inport
  Gain : Gain  Gain=0.2951
  Integrator : Integrator  InitialCondition=13.359685039370081  LimitOutput=on  UpperSaturationLimit=15.07125  LowerSaturationLimit=10
  Out1 : Outport
  wires:
  In1/1 -> Gain/1
  Gain/1 -> Integrator/1
  Integrator/1 -> Out1/1

== system sm_boom_lift_crawler_abstract_flex_boom/Abstract Actuators/Logic to p OutFR ==
  In1 : Inport
  Gain : Gain  Gain=0.2951
  Integrator : Integrator  InitialCondition=13.359685039370081  LimitOutput=on  UpperSaturationLimit=15.07125  LowerSaturationLimit=10
  Out1 : Outport
  wires:
  Gain/1 -> Integrator/1
  In1/1 -> Gain/1
  Integrator/1 -> Out1/1

== system sm_boom_lift_crawler_abstract_flex_boom/Abstract Actuators/Logic to p OutRL ==
  In1 : Inport
  Gain : Gain  Gain=0.2917
  Integrator : Integrator  InitialCondition=13.004645669291337  LimitOutput=on  UpperSaturationLimit=14.69659  LowerSaturationLimit=10
  Out1 : Outport
  wires:
  Gain/1 -> Integrator/1
  In1/1 -> Gain/1
  Integrator/1 -> Out1/1

== system sm_boom_lift_crawler_abstract_flex_boom/Abstract Actuators/Logic to p OutRR ==
  In1 : Inport
  Gain : Gain  Gain=0.2911
  Integrator : Integrator  InitialCondition=13.207637795275589  LimitOutput=on  UpperSaturationLimit=14.89625  LowerSaturationLimit=10
  Out1 : Outport
  wires:
  Gain/1 -> Integrator/1
  In1/1 -> Gain/1
  Integrator/1 -> Out1/1

== system sm_boom_lift_crawler_abstract_flex_boom/Abstract Actuators/Logic to p Tilt ==
  In1 : Inport
  Gain : Gain  Gain=0.0139
  Integrator : Integrator  LimitOutput=on  UpperSaturationLimit=0.57  LowerSaturationLimit=0
  Out1 : Outport
  wires:
  Integrator/1 -> Out1/1
  In1/1 -> Gain/1
  Gain/1 -> Integrator/1

== system sm_boom_lift_crawler_abstract_flex_boom/Abstract Actuators/Logic to p TrackL ==
  In1 : Inport
  Gain : Gain  Gain=1/7
  Integrator : Integrator  LimitOutput=on  UpperSaturationLimit=0.305  LowerSaturationLimit=0
  Out1 : Outport
  wires:
  In1/1 -> Gain/1
  Integrator/1 -> Out1/1
  Gain/1 -> Integrator/1

== system sm_boom_lift_crawler_abstract_flex_boom/Abstract Actuators/Logic to p TrackR ==
  In1 : Inport
  Gain : Gain  Gain=1/7
  Integrator : Integrator  LimitOutput=on  UpperSaturationLimit=0.305  LowerSaturationLimit=0
  Out1 : Outport
  wires:
  Gain/1 -> Integrator/1
  Integrator/1 -> Out1/1
  In1/1 -> Gain/1

== system sm_boom_lift_crawler_abstract_flex_boom/Abstract Actuators/Logic to q Turret ==
  In1 : Inport
  Gain : Gain  Gain=158.9/25.5
  Integrator : Integrator  LimitOutput=on  UpperSaturationLimit=158.9  LowerSaturationLimit=-158.9
  Scope : Scope  NumInputPorts=2
      settings: ActiveDisplayYMinimum=-1.25  ActiveDisplayYMaximum=1.25  DataLoggingVariableName=ScopeData3
  Out1 : Outport
  wires:
  Integrator/1 -> Scope/2, Out1/1
  In1/1 -> Scope/1, Gain/1
  Gain/1 -> Integrator/1

== system sm_boom_lift_crawler_abstract_flex_boom/Control/Direct ==
  O : Inport
  M : Inport  Port=2
  Bus Creator : BusCreator  Inputs=1
  Constant : Constant
  Terminator1 : Terminator
  S : Outport
  A : Outport  Port=2
  wires:
  M/1 -> Terminator1/1
  O/1 -> A/1
  Bus Creator/1 -> S/1
  Constant/1 -> Bus Creator/1  "Jib Align"

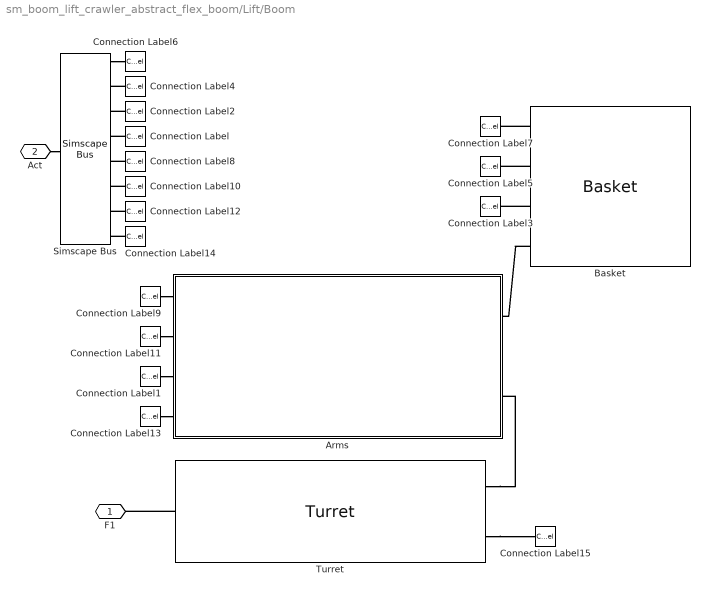
== system sm_boom_lift_crawler_abstract_flex_boom/Lift/Boom ==
  Arms : Subsystem
      mask Display: image('sm002_trim_arm_telescope.svg')
  Basket : sm_boom_lift_crawler_lib_boom/Boom/Basket  SystemSampleTime=-1  VariantActivationTime=update diagram  EmptyChoice=off  PassThrough=off  PassThroughVariantControl=(default)  EmptyChoiceVariantControl=(default)  AllowFlexibleInterface=on  Latency=0  AutoFrameSizeCalculation=off
  Connection Label : ConnectionLabel  Label=Tilt
  Connection Label1 : ConnectionLabel  Label=Tilt
  Connection Label10 : ConnectionLabel  Label=LevelM
  Connection Label11 : ConnectionLabel  Label=LevelM
  Connection Label12 : ConnectionLabel  Label=Lift
  Connection Label13 : ConnectionLabel  Label=Lift
  Connection Label14 : ConnectionLabel  Label=Turret
  Connection Label15 : ConnectionLabel  Label=Turret
  Connection Label2 : ConnectionLabel  Label=Jib
  Connection Label3 : ConnectionLabel  Label=Jib
  Connection Label4 : ConnectionLabel  Label=BasketR
  Connection Label5 : ConnectionLabel  Label=BasketR
  Connection Label6 : ConnectionLabel  Label=LevelS
  Connection Label7 : ConnectionLabel  Label=LevelS
  Connection Label8 : ConnectionLabel  Label=Extend
  Connection Label9 : ConnectionLabel  Label=Extend
  Simscape Bus : SimscapeBus  HierarchyStrings=LevelS;BasketR;Jib;Tilt;Extend;LevelM;Lift;Turret
  Turret : sm_boom_lift_crawler_lib_boom/Boom/Turret  SystemSampleTime=-1  VariantActivationTime=update diagram  EmptyChoice=off  PassThrough=off  PassThroughVariantControl=(default)  EmptyChoiceVariantControl=(default)  AllowFlexibleInterface=on  Latency=0  AutoFrameSizeCalculation=off
  F1 : PMIOPort  Side=Right
  Act : PMIOPort  Port=2  Side=Left
  connections:
  Turret/LConn1 -- F1/RConn1
  Connection Label/LConn1 -- Simscape Bus/LConn4
  Act/RConn1 -- Simscape Bus/RConn1
  Connection Label2/LConn1 -- Simscape Bus/LConn3
  Basket/RConn3 -- Connection Label3/LConn1
  Connection Label4/LConn1 -- Simscape Bus/LConn2
  Basket/RConn2 -- Connection Label5/LConn1
  Simscape Bus/LConn1 -- Connection Label6/LConn1
  Basket/RConn1 -- Connection Label7/LConn1
  Connection Label8/LConn1 -- Simscape Bus/LConn5
  Connection Label10/LConn1 -- Simscape Bus/LConn6
  Connection Label12/LConn1 -- Simscape Bus/LConn7
  Connection Label14/LConn1 -- Simscape Bus/LConn8
  Turret/RConn2 -- Connection Label15/LConn1
  Basket/RConn4 -- Arms/RConn1
  Connection Label9/LConn1 -- Arms/LConn1
  Connection Label11/LConn1 -- Arms/LConn2
  Connection Label1/LConn1 -- Arms/LConn3
  Connection Label13/LConn1 -- Arms/LConn4
  Turret/RConn1 -- Arms/RConn2

== system sm_boom_lift_crawler_abstract_flex_boom/Lift/Ground Contact Pads ==
  Constraint : Subsystem  VariantControl=Constraint
      mask Display: image('sm_boom_lift_crawler_outr_floor_constraint.svg');
  Force : Subsystem  VariantControl=Force
      mask Display: image('sm_boom_lift_crawler_contact_outr_floor.svg');
  RL : PMIOPort  Side=Right
  RR : PMIOPort  Port=2  Side=Right
  FR : PMIOPort  Port=3  Side=Right
  FL : PMIOPort  Port=4  Side=Right
  RLb : PMIOPort  Port=5  Side=Left
  RRb : PMIOPort  Port=6  Side=Left
  FRb : PMIOPort  Port=7  Side=Left
  FLb : PMIOPort  Port=8  Side=Left
